simulink model "LQR_Blank"  (R2017b)
settings: Solver=FixedStepAuto  StartTime=0.0  StopTime=25  FixedStep=0.001  RelTol=1e-3
model workspace (MAT data in the model file):
  Af = 0.027
  Cd = 32.3127
  Q = 1
  R = 1
  Rx = 1.6517
  Tf = 25
  g = 9.81
  height = 0.12
  m = 3
  rho = 1.225
  v = 0
  width = 0.25
values from neighbouring files (symbols this model uses):
  A_f = 1.6 + 0.00056*(m - 765)    [ME_131_HW5.m]    (also in ME_131_Lab6.m = 0.03375)
  C_d = (2*m*beta*atan(beta)) / (V_o*T*rho*A_f)    [ME_131_HW5.m]    (also in ME_131_Lab6.m = 9.0138)
  K = lqr(A,B,Q,R)    [ME_131_Lab6.m]
  R_x = (V_o*m*atan(beta)) / (beta*T)    [ME_131_HW5.m]    (also in ME_131_Lab6.m = 8.2029)
  V_init = 0.5    [ME_131_Lab6.m]
settings Model: Creator=vallon2  LastModifiedBy=sachi

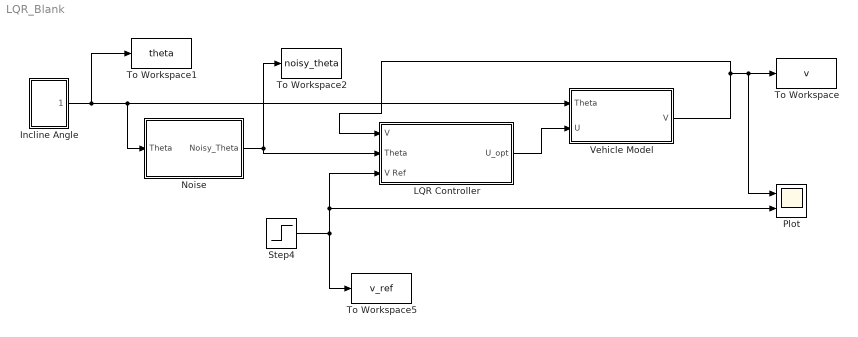
== system LQR_Blank ==
  Incline Angle : Subsystem
  LQR Controller : Subsystem
  "Noise " : Subsystem
  "Plot " : Scope  NumInputPorts=2
  Step4 : Step  Time=10  Before=0.5  SampleTime=0
  To Workspace : ToWorkspace  VariableName=v  SaveFormat=Timeseries  SampleTime=-1
  To Workspace1 : ToWorkspace  VariableName=theta  SaveFormat=Timeseries  SampleTime=-1
  To Workspace2 : ToWorkspace  VariableName=noisy_theta  SaveFormat=Timeseries  SampleTime=-1
  To Workspace5 : ToWorkspace  VariableName=v_ref  SaveFormat=Timeseries  SampleTime=-1
  Vehicle Model : Subsystem
  wires:
  Step4/1 -> To Workspace5/1, "Plot "/2, LQR Controller/3(V Ref)
  Vehicle Model/1(V) -> To Workspace/1, "Plot "/1, LQR Controller/1("V ")
  LQR Controller/1("U_opt ") -> Vehicle Model/2(U)
  "Noise "/1("Noisy_Theta ") -> LQR Controller/2(Theta), To Workspace2/1
  Incline Angle/1("Theta ") -> To Workspace1/1, Vehicle Model/1(Theta), "Noise "/1("Theta ")

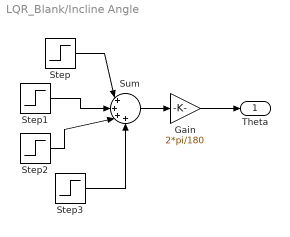
== system LQR_Blank/Incline Angle ==
  Gain : Gain  Gain=2*pi/180
  Step : Step  Time=3  After=10  SampleTime=0
  Step1 : Step  Time=8  After=10  SampleTime=0
  Step2 : Step  Time=13  After=-35  SampleTime=0
  Step3 : Step  Time=17  After=15  SampleTime=0
  Sum : Sum  Inputs=|++++
  "Theta " : Outport
  wires:
  Step/1 -> Sum/1
  Step1/1 -> Sum/2
  Step3/1 -> Sum/4
  Sum/1 -> Gain/1
  Gain/1 -> "Theta "/1
  Step2/1 -> Sum/3

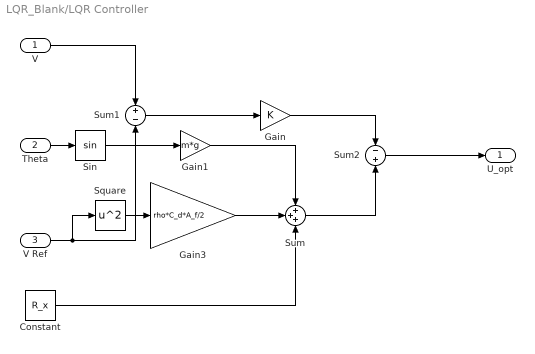
== system LQR_Blank/LQR Controller ==
  "V " : Inport
  Theta : Inport  Port=2
  V Ref : Inport  Port=3
  Constant : Constant  Value=R_x
  Gain : Gain  Gain=K
  Gain1 : Gain  Gain=m*g
  Gain3 : Gain  Gain=rho*C_d*A_f/2
  Sin : Trigonometry
  Square : Math  Operator=square  RndMeth=Zero  SaturateOnIntegerOverflow=on
  Sum : Sum  Inputs=+++
  Sum1 : Sum  Inputs=+-
  Sum2 : Sum  Inputs=-+
  "U_opt " : Outport
  wires:
  Theta/1 -> Sin/1
  Constant/1 -> Sum/3
  "V "/1 -> Sum1/1
  V Ref/1 -> Sum1/2, Square/1
  Sum1/1 -> Gain/1
  Gain/1 -> Sum2/1
  Sum/1 -> Sum2/2
  Sum2/1 -> "U_opt "/1
  Sin/1 -> Gain1/1
  Gain1/1 -> Sum/1
  Square/1 -> Gain3/1
  Gain3/1 -> Sum/2

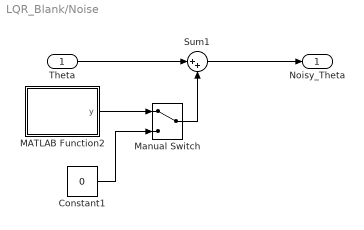
== system LQR_Blank/Noise  ==
  "Theta " : Inport
  Constant1 : Constant  Value=0
  MATLAB Function2 : MATLAB Function  TreatAsAtomicUnit=on
  Manual Switch : ManualSwitch
  Sum1 : Sum  Inputs=|++
  "Noisy_Theta " : Outport
  wires:
  Constant1/1 -> Manual Switch/2
  Sum1/1 -> "Noisy_Theta "/1
  MATLAB Function2/1(y) -> Manual Switch/1
  "Theta "/1 -> Sum1/1
  Manual Switch/1 -> Sum1/2

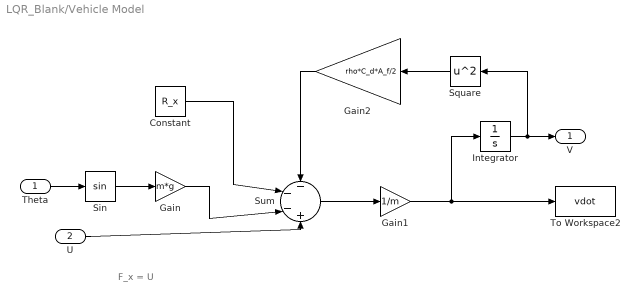
== system LQR_Blank/Vehicle Model ==
  note: F_x = U
  Theta : Inport
  U : Inport  Port=2
  Constant : Constant  Value=R_x
  Gain : Gain  Gain=m*g
  Gain1 : Gain  Gain=1/m
  Gain2 : Gain  Gain=rho*C_d*A_f/2
  Integrator : Integrator  InitialCondition=V_init
  Sin : Trigonometry
  Square : Math  Operator=square  RndMeth=Zero  SaturateOnIntegerOverflow=on
  Sum : Sum  Inputs=---+
  To Workspace2 : ToWorkspace  VariableName=vdot  SaveFormat=Timeseries  SampleTime=-1
  V : Outport
  wires:
  Theta/1 -> Sin/1
  Sin/1 -> Gain/1
  Constant/1 -> Sum/2
  Gain/1 -> Sum/3
  U/1 -> Sum/4
  Sum/1 -> Gain1/1
  Gain1/1 -> Integrator/1, To Workspace2/1
  Integrator/1 -> Square/1, V/1
  Square/1 -> Gain2/1
  Gain2/1 -> Sum/1

== matlab function LQR_Blank/Noise /MATLAB Function2 ==
  data: y output
function y = noise
y = 0.01*randn(1);
